simulink library "acm_lookup_generic_relay"  (Simulink 7.6)
settings: Solver=ode45  SolverMode=SingleTasking  StartTime=0.0  StopTime=10.0  RelTol=1e-3
undefined symbols (not defined in the file): sMP
settings Model: Creator=RAFREY5  LastModifiedBy=aoverfe

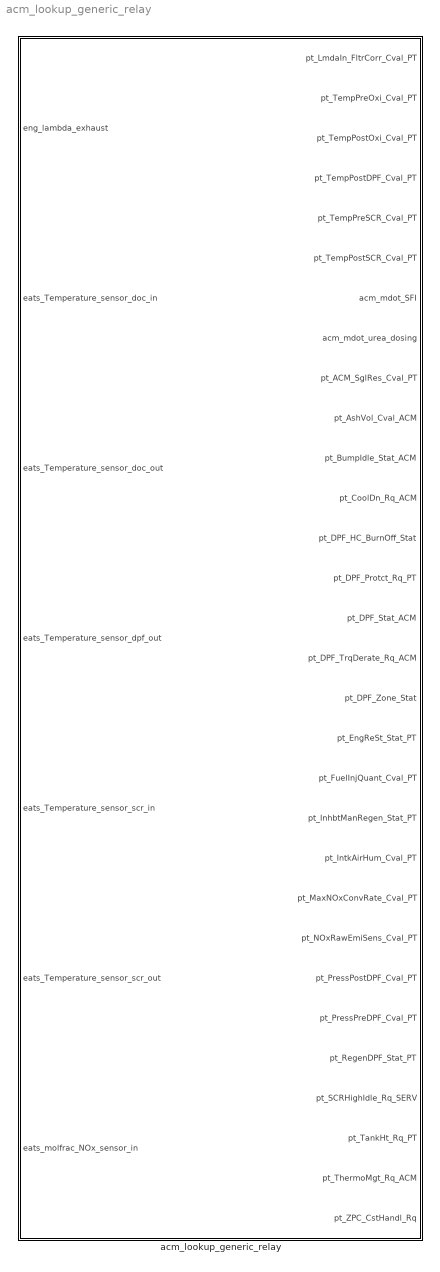
== system acm_lookup_generic_relay ==
  acm_lookup_generic_relay : Subsystem  mask(DIVeMB lookup){acm_mdot_SFI=sMP.ctrl.acm.out.acm_mdot_SFI, acm_mdot_urea_dosing=sMP.ctrl.acm.out.acm_mdot_urea_dosing, pt_ACM_SglRes_Cval_PT=sMP.ctrl.acm.out.pt_ACM_SglRes_Cval_PT, pt_AshVol_Cval_ACM=sMP.ctrl.acm.out.pt_AshVol_Cval_ACM, pt_BumpIdle_Stat_ACM=sMP.ctrl.acm.out.pt_BumpIdle_Stat_ACM, pt_CoolDn_Rq_ACM=sMP.ctrl.acm.out.pt_CoolDn_Rq_ACM, pt_DPF_HC_BurnOff_Stat=sMP.ctrl.acm.out.pt_DPF_HC_BurnOff_Stat, pt_DPF_Protct_Rq_PT=sMP.ctrl.acm.out.pt_DPF_Protct_Rq_PT, pt_DPF_Stat_ACM=sMP.ctrl.acm.out.pt_DPF_Stat_ACM, pt_DPF_TrqDerate_Rq_ACM=sMP.ctrl.acm.out.pt_DPF_TrqDerate_Rq_ACM, pt_DPF_Zone_Stat=sMP.ctrl.acm.out.pt_DPF_Zone_Stat, pt_EngReSt_Stat_PT=sMP.ctrl.acm.out.pt_EngReSt_Stat_PT, pt_FuelInjQuant_Cval_PT=sMP.ctrl.acm.out.pt_FuelInjQuant_Cval_PT, pt_InhbtManRegen_Stat_PT=sMP.ctrl.acm.out.pt_InhbtManRegen_Stat_PT, pt_IntkAirHum_Cval_PT=sMP.ctrl.acm.out.pt_IntkAirHum_Cval_PT, pt_MaxNOxConvRate_Cval_PT=sMP.ctrl.acm.out.pt_MaxNOxConvRate_Cval_PT, pt_NOxRawEmiSens_Cval_PT=sMP.ctrl.acm.out.pt_NOxRawEmiSens_Cval_PT, pt_PressPostDPF_Cval_PT=sMP.ctrl.acm.out.pt_PressPostDPF_Cval_PT, pt_PressPreDPF_Cval_PT=sMP.ctrl.acm.out.pt_PressPreDPF_Cval_PT, pt_RegenDPF_Stat_PT=sMP.ctrl.acm.out.pt_RegenDPF_Stat_PT, pt_SCRHighIdle_Rq_SERV=sMP.ctrl.acm.out.pt_SCRHighIdle_Rq_SERV, pt_TankHt_Rq_PT=sMP.ctrl.acm.out.pt_TankHt_Rq_PT, pt_ThermoMgt_Rq_ACM=sMP.ctrl.acm.out.pt_ThermoMgt_Rq_ACM, pt_ZPC_CstHandl_Rq=sMP.ctrl.acm.out.pt_ZPC_CstHandl_Rq}
      mask prompts: acm_mdot_SFI "Massflow of secondary fuel injection (before DOC) (constant) [g/s]"; acm_mdot_urea_dosing "Massflow of urea/AdBlue (constant) [g/h]"; pt_ACM_SglRes_Cval_PT "Constant value of pt_ACM_SglRes_Cval_PT"; pt_AshVol_Cval_ACM "Constant value of  pt_AshVol_Cval_ACM"; pt_BumpIdle_Stat_ACM "Constant value of pt_BumpIdle_Stat_ACM"; pt_CoolDn_Rq_ACM "Constant value of pt_CoolDn_Rq_ACM"; pt_DPF_HC_BurnOff_Stat "Constant value of pt_DPF_HC_BurnOff_Stat"; pt_DPF_Protct_Rq_PT "Constant value of pt_DPF_Protct_Rq_PT"; pt_DPF_Stat_ACM "Constant value of pt_DPF_Stat_ACM"; pt_DPF_TrqDerate_Rq_ACM "Constant value of pt_DPF_TrqDerate_Rq_ACM"; pt_DPF_Zone_Stat "Constant value of pt_DPF_Zone_Stat"; pt_EngReSt_Stat_PT "Constant value of pt_EngReSt_Stat_PT"; pt_FuelInjQuant_Cval_PT "Constant value of pt_FuelInjQuant_Cval_PT"; pt_InhbtManRegen_Stat_PT "Constant value of pt_InhbtManRegen_Stat_PT"; pt_IntkAirHum_Cval_PT "Constant value of pt_IntkAirHum_Cval_PT"; pt_MaxNOxConvRate_Cval_PT "Constant value of pt_MaxNOxConvRate_Cval_PT"; pt_NOxRawEmiSens_Cval_PT "Constant value of pt_NOxRawEmiSens_Cval_PT"; pt_PressPostDPF_Cval_PT "Constant value of pt_PressPostDPF_Cval_PT"; pt_PressPreDPF_Cval_PT "Constant value of pt_PressPreDPF_Cval_PT"; pt_RegenDPF_Stat_PT "Constant value of pt_RegenDPF_Stat_PT"; pt_SCRHighIdle_Rq_SERV "Constant value of pt_SCRHighIdle_Rq_SERV"; pt_TankHt_Rq_PT "Constant value of pt_TankHt_Rq_PT"; pt_ThermoMgt_Rq_ACM "Constant value of pt_ThermoMgt_Rq_ACM"; pt_ZPC_CstHandl_Rq "Constant value of pt_ZPC_CstHandl_Rq"
      mask help:
      | This block relays signals of engine and EATS to allow a correct MCM operation for thermomanagent map determination according EATS temperatures and NOx sensor signal without an real ACM.
      |
      | The SFI and urea dosing values are only constant signals to satisfy special MCM instruemantion blocks (OutputMVA).

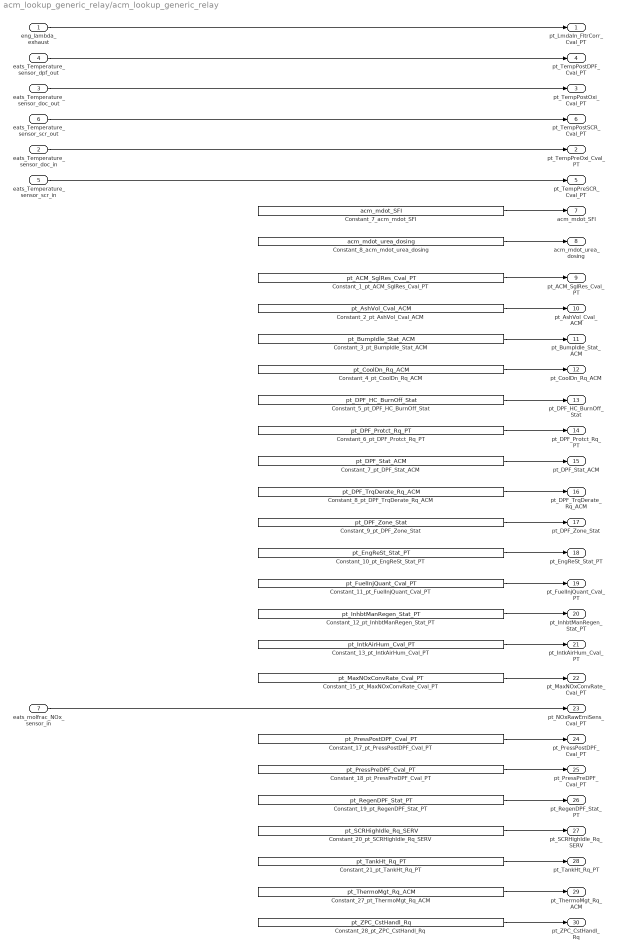
== system acm_lookup_generic_relay/acm_lookup_generic_relay ==
  eng_lambda_exhaust : Inport
  eats_Temperature_sensor_doc_in : Inport  Port=2
  eats_Temperature_sensor_doc_out : Inport  Port=3
  eats_Temperature_sensor_dpf_out : Inport  Port=4
  eats_Temperature_sensor_scr_in : Inport  Port=5
  eats_Temperature_sensor_scr_out : Inport  Port=6
  eats_molfrac_NOx_sensor_in : Inport  Port=7
  Constant_10_pt_EngReSt_Stat_PT : Constant  Value=pt_EngReSt_Stat_PT
  Constant_11_pt_FuelInjQuant_Cval_PT : Constant  Value=pt_FuelInjQuant_Cval_PT
  Constant_12_pt_InhbtManRegen_Stat_PT : Constant  Value=pt_InhbtManRegen_Stat_PT
  Constant_13_pt_IntkAirHum_Cval_PT : Constant  Value=pt_IntkAirHum_Cval_PT
  Constant_15_pt_MaxNOxConvRate_Cval_PT : Constant  Value=pt_MaxNOxConvRate_Cval_PT
  Constant_17_pt_PressPostDPF_Cval_PT : Constant  Value=pt_PressPostDPF_Cval_PT
  Constant_18_pt_PressPreDPF_Cval_PT : Constant  Value=pt_PressPreDPF_Cval_PT
  Constant_19_pt_RegenDPF_Stat_PT : Constant  Value=pt_RegenDPF_Stat_PT
  Constant_1_pt_ACM_SglRes_Cval_PT : Constant  Value=pt_ACM_SglRes_Cval_PT
  Constant_20_pt_SCRHighIdle_Rq_SERV : Constant  Value=pt_SCRHighIdle_Rq_SERV
  Constant_21_pt_TankHt_Rq_PT : Constant  Value=pt_TankHt_Rq_PT
  Constant_27_pt_ThermoMgt_Rq_ACM : Constant  Value=pt_ThermoMgt_Rq_ACM
  Constant_28_pt_ZPC_CstHandl_Rq : Constant  Value=pt_ZPC_CstHandl_Rq
  Constant_2_pt_AshVol_Cval_ACM : Constant  Value=pt_AshVol_Cval_ACM
  Constant_3_pt_BumpIdle_Stat_ACM : Constant  Value=pt_BumpIdle_Stat_ACM
  Constant_4_pt_CoolDn_Rq_ACM : Constant  Value=pt_CoolDn_Rq_ACM
  Constant_5_pt_DPF_HC_BurnOff_Stat : Constant  Value=pt_DPF_HC_BurnOff_Stat
  Constant_6_pt_DPF_Protct_Rq_PT : Constant  Value=pt_DPF_Protct_Rq_PT
  Constant_7_acm_mdot_SFI : Constant  Value=acm_mdot_SFI
  Constant_7_pt_DPF_Stat_ACM : Constant  Value=pt_DPF_Stat_ACM
  Constant_8_acm_mdot_urea_dosing : Constant  Value=acm_mdot_urea_dosing
  Constant_8_pt_DPF_TrqDerate_Rq_ACM : Constant  Value=pt_DPF_TrqDerate_Rq_ACM
  Constant_9_pt_DPF_Zone_Stat : Constant  Value=pt_DPF_Zone_Stat
  pt_LmdaIn_FltrCorr_Cval_PT : Outport
  pt_TempPreOxi_Cval_PT : Outport  Port=2
  pt_TempPostOxi_Cval_PT : Outport  Port=3
  pt_TempPostDPF_Cval_PT : Outport  Port=4
  pt_TempPreSCR_Cval_PT : Outport  Port=5
  pt_TempPostSCR_Cval_PT : Outport  Port=6
  acm_mdot_SFI : Outport  Port=7
  acm_mdot_urea_dosing : Outport  Port=8
  pt_ACM_SglRes_Cval_PT : Outport  Port=9
  pt_AshVol_Cval_ACM : Outport  Port=10
  pt_BumpIdle_Stat_ACM : Outport  Port=11
  pt_CoolDn_Rq_ACM : Outport  Port=12
  pt_DPF_HC_BurnOff_Stat : Outport  Port=13
  pt_DPF_Protct_Rq_PT : Outport  Port=14
  pt_DPF_Stat_ACM : Outport  Port=15
  pt_DPF_TrqDerate_Rq_ACM : Outport  Port=16
  pt_DPF_Zone_Stat : Outport  Port=17
  pt_EngReSt_Stat_PT : Outport  Port=18
  pt_FuelInjQuant_Cval_PT : Outport  Port=19
  pt_InhbtManRegen_Stat_PT : Outport  Port=20
  pt_IntkAirHum_Cval_PT : Outport  Port=21
  pt_MaxNOxConvRate_Cval_PT : Outport  Port=22
  pt_NOxRawEmiSens_Cval_PT : Outport  Port=23
  pt_PressPostDPF_Cval_PT : Outport  Port=24
  pt_PressPreDPF_Cval_PT : Outport  Port=25
  pt_RegenDPF_Stat_PT : Outport  Port=26
  pt_SCRHighIdle_Rq_SERV : Outport  Port=27
  pt_TankHt_Rq_PT : Outport  Port=28
  pt_ThermoMgt_Rq_ACM : Outport  Port=29
  pt_ZPC_CstHandl_Rq : Outport  Port=30
  wires:
  eats_Temperature_sensor_doc_in/1 -> pt_TempPreOxi_Cval_PT/1
  eng_lambda_exhaust/1 -> pt_LmdaIn_FltrCorr_Cval_PT/1
  eats_Temperature_sensor_dpf_out/1 -> pt_TempPostDPF_Cval_PT/1
  eats_Temperature_sensor_doc_out/1 -> pt_TempPostOxi_Cval_PT/1
  eats_Temperature_sensor_scr_out/1 -> pt_TempPostSCR_Cval_PT/1
  eats_Temperature_sensor_scr_in/1 -> pt_TempPreSCR_Cval_PT/1
  Constant_7_acm_mdot_SFI/1 -> acm_mdot_SFI/1
  Constant_8_acm_mdot_urea_dosing/1 -> acm_mdot_urea_dosing/1
  Constant_1_pt_ACM_SglRes_Cval_PT/1 -> pt_ACM_SglRes_Cval_PT/1
  Constant_2_pt_AshVol_Cval_ACM/1 -> pt_AshVol_Cval_ACM/1
  Constant_3_pt_BumpIdle_Stat_ACM/1 -> pt_BumpIdle_Stat_ACM/1
  Constant_4_pt_CoolDn_Rq_ACM/1 -> pt_CoolDn_Rq_ACM/1
  Constant_5_pt_DPF_HC_BurnOff_Stat/1 -> pt_DPF_HC_BurnOff_Stat/1
  Constant_6_pt_DPF_Protct_Rq_PT/1 -> pt_DPF_Protct_Rq_PT/1
  Constant_7_pt_DPF_Stat_ACM/1 -> pt_DPF_Stat_ACM/1
  Constant_8_pt_DPF_TrqDerate_Rq_ACM/1 -> pt_DPF_TrqDerate_Rq_ACM/1
  Constant_9_pt_DPF_Zone_Stat/1 -> pt_DPF_Zone_Stat/1
  Constant_10_pt_EngReSt_Stat_PT/1 -> pt_EngReSt_Stat_PT/1
  Constant_11_pt_FuelInjQuant_Cval_PT/1 -> pt_FuelInjQuant_Cval_PT/1
  Constant_12_pt_InhbtManRegen_Stat_PT/1 -> pt_InhbtManRegen_Stat_PT/1
  Constant_13_pt_IntkAirHum_Cval_PT/1 -> pt_IntkAirHum_Cval_PT/1
  Constant_15_pt_MaxNOxConvRate_Cval_PT/1 -> pt_MaxNOxConvRate_Cval_PT/1
  eats_molfrac_NOx_sensor_in/1 -> pt_NOxRawEmiSens_Cval_PT/1
  Constant_17_pt_PressPostDPF_Cval_PT/1 -> pt_PressPostDPF_Cval_PT/1
  Constant_18_pt_PressPreDPF_Cval_PT/1 -> pt_PressPreDPF_Cval_PT/1
  Constant_19_pt_RegenDPF_Stat_PT/1 -> pt_RegenDPF_Stat_PT/1
  Constant_20_pt_SCRHighIdle_Rq_SERV/1 -> pt_SCRHighIdle_Rq_SERV/1
  Constant_21_pt_TankHt_Rq_PT/1 -> pt_TankHt_Rq_PT/1
  Constant_27_pt_ThermoMgt_Rq_ACM/1 -> pt_ThermoMgt_Rq_ACM/1
  Constant_28_pt_ZPC_CstHandl_Rq/1 -> pt_ZPC_CstHandl_Rq/1
